simulink model "SUBS_CARGA"  (R2024b)
settings: Solver=VariableStepAuto  StartTime=0.0  StopTime=10.0  RelTol=1e-3
undefined symbols (not defined in the file): bcx, bcy, dx_l_ini, dy_l_ini, g, Hc, Kcy, M_x, Ms, x_l_ini, y_l_ini
settings Model: Creator=ribei  LastModifiedBy=ribei

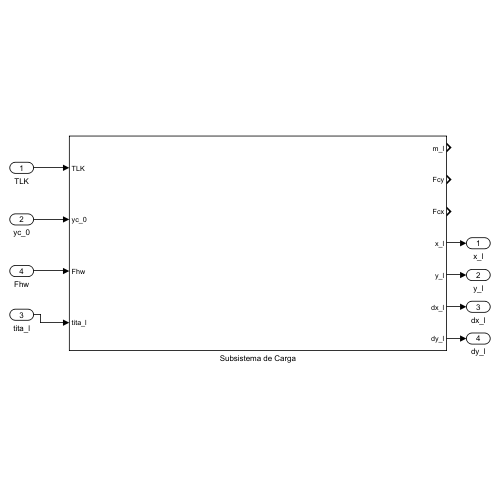
[thumbnail: Simulink's stored preview of the top-level diagram]
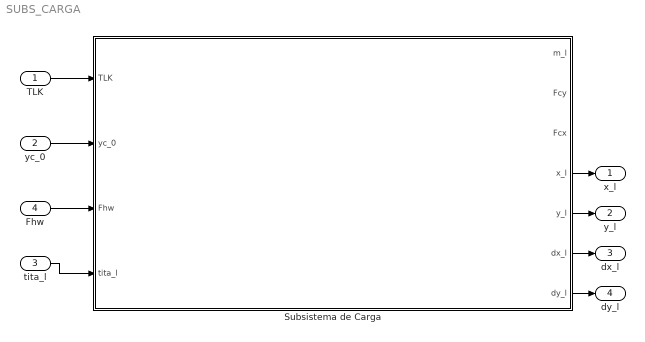
== system SUBS_CARGA ==
  TLK : Inport
  yc_0 : Inport  Port=2
  tita_l : Inport  Port=3
  Fhw : Inport  Port=4
  Subsistema de Carga : Subsystem
  x_l : Outport
  y_l : Outport  Port=2
  dx_l : Outport  Port=3
  dy_l : Outport  Port=4
  wires:
  TLK/1 -> Subsistema de Carga/1(TLK)
  yc_0/1 -> Subsistema de Carga/2(yc_0)
  Fhw/1 -> Subsistema de Carga/3(Fhw)
  tita_l/1 -> Subsistema de Carga/4(tita_l)
  Subsistema de Carga/4(x_l) -> x_l/1
  Subsistema de Carga/5(y_l) -> y_l/1
  Subsistema de Carga/6(dx_l) -> dx_l/1
  Subsistema de Carga/7(dy_l) -> dy_l/1

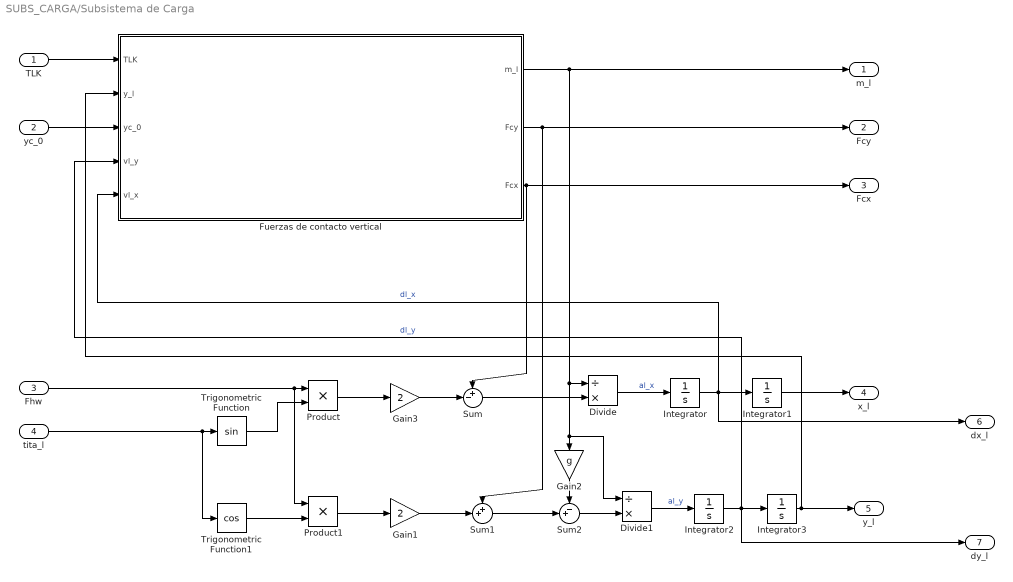
== system SUBS_CARGA/Subsistema de Carga ==
  TLK : Inport
  yc_0 : Inport  Port=2
  Fhw : Inport  Port=3
  tita_l : Inport  Port=4
  Divide : Product  Inputs=/*
  Divide1 : Product  Inputs=/*
  Fuerzas de contacto vertical : Subsystem
  Gain1 : Gain  Gain=2
  Gain2 : Gain  Gain=g
  Gain3 : Gain  Gain=2
  Integrator : Integrator  InitialCondition=dx_l_ini
  Integrator1 : Integrator  InitialCondition=x_l_ini
  Integrator2 : Integrator  InitialCondition=dy_l_ini
  Integrator3 : Integrator  InitialCondition=y_l_ini
  Product : Product
  Product1 : Product
  Sum : Sum  Inputs=+-|
  Sum1 : Sum  Inputs=++|
  Sum2 : Sum  Inputs=-+|
  Trigonometric Function : Trigonometry
  Trigonometric Function1 : Trigonometry  Operator=cos
  m_l : Outport
  Fcy : Outport  Port=2
  Fcx : Outport  Port=3
  x_l : Outport  Port=4
  y_l : Outport  Port=5
  dx_l : Outport  Port=6
  dy_l : Outport  Port=7
  wires:
  Fuerzas de contacto vertical/1(m_l) -> m_l/1, Divide/1, Divide1/1, Gain2/1
  Fuerzas de contacto vertical/3(Fcx) -> Fcx/1, Sum/1
  Integrator3/1 -> y_l/1, Fuerzas de contacto vertical/2(y_l)
  Divide1/1 -> Integrator2/1  "al_y"
  Sum/1 -> Divide/2
  Gain1/1 -> Sum1/2
  Divide/1 -> Integrator/1  "al_x"
  Integrator2/1 -> Integrator3/1, dy_l/1, Fuerzas de contacto vertical/4(vl_y)  "dl_y"
  Sum1/1 -> Sum2/2
  tita_l/1 -> Trigonometric Function1/1, Trigonometric Function/1
  Product1/1 -> Gain1/1
  Integrator/1 -> Fuerzas de contacto vertical/5(vl_x), Integrator1/1, dx_l/1  "dl_x"
  Trigonometric Function/1 -> Product/2
  Fuerzas de contacto vertical/2(Fcy) -> Fcy/1, Sum1/1
  Product/1 -> Gain3/1
  Gain3/1 -> Sum/2
  Sum2/1 -> Divide1/2
  Fhw/1 -> Product1/1, Product/1
  Trigonometric Function1/1 -> Product1/2
  Gain2/1 -> Sum2/1
  TLK/1 -> Fuerzas de contacto vertical/1(TLK)
  yc_0/1 -> Fuerzas de contacto vertical/3(yc_0)
  Integrator1/1 -> x_l/1

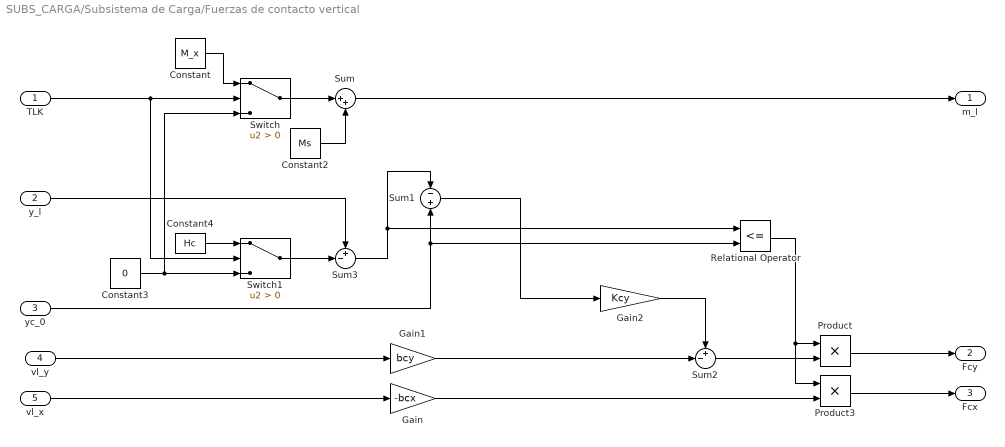
== system SUBS_CARGA/Subsistema de Carga/Fuerzas de contacto vertical ==
  TLK : Inport
  y_l : Inport  Port=2
  yc_0 : Inport  Port=3
  vl_y : Inport  Port=4
  vl_x : Inport  Port=5
  Constant : Constant  Value=M_x
  Constant2 : Constant  Value=Ms
  Constant3 : Constant  Value=0
  Constant4 : Constant  Value=Hc
  Gain : Gain  Gain=-bcx
  Gain1 : Gain  Gain=bcy
  Gain2 : Gain  Gain=Kcy
  Product : Product
  Product3 : Product
  Relational Operator : RelationalOperator  Operator=<=  OutDataTypeStr=boolean  RndMeth=Simplest  InputSameDT=off
  Sum : Sum  Inputs=|++
  Sum1 : Sum  Inputs=-|+
  Sum2 : Sum  Inputs=+-|
  Sum3 : Sum  Inputs=+-|
  Switch : Switch  Criteria=u2 > Threshold  SaturateOnIntegerOverflow=off  InputSameDT=off
  Switch1 : Switch  Criteria=u2 > Threshold  SaturateOnIntegerOverflow=off  InputSameDT=off
  m_l : Outport
  Fcy : Outport  Port=2
  Fcx : Outport  Port=3
  wires:
  TLK/1 -> Switch/2, Switch1/2
  Gain1/1 -> Sum2/2
  Switch/1 -> Sum/1
  Constant3/1 -> Switch1/3, Switch/3
  yc_0/1 -> Relational Operator/2, Sum1/2
  Constant2/1 -> Sum/2
  Sum3/1 -> Relational Operator/1, Sum1/1
  Sum2/1 -> Product/2
  vl_y/1 -> Gain1/1
  Gain/1 -> Product3/2
  Switch1/1 -> Sum3/2
  Constant4/1 -> Switch1/1
  vl_x/1 -> Gain/1
  Gain2/1 -> Sum2/1
  Sum1/1 -> Gain2/1
  Sum/1 -> m_l/1
  y_l/1 -> Sum3/1
  Constant/1 -> Switch/1
  Product/1 -> Fcy/1
  Product3/1 -> Fcx/1
  Relational Operator/1 -> Product3/1, Product/1
